simulink model "Model2_2023b"  (R2023b)
settings: Solver=ode4  StartTime=0.0  StopTime=100  FixedStep=0.01  RelTol=1e-3
values from neighbouring files (symbols this model uses):
  ARM_P_PID = [10 0 20]*0.1    [Single_ARM_Monte.m]    (also in main_starter.m)
  ARM_T_PID = [100 0 0]    [Single_ARM_Monte.m]    (also in main_starter.m)
  ARM_V_PID = [10 0 5]*0.1    [Single_ARM_Monte.m]    (also in main_starter.m)
  D_Joint0_angle0 = 45    [Single_ARM_Monte.m]    (also in main_starter.m)
  D_Joint0_angle1 = 0    [Single_ARM_Monte.m]    (also in main_starter.m)
  D_Joint0_angle2 = 0    [Single_ARM_Monte.m]    (also in main_starter.m)
  D_Joint0_rate0 = 0    [Single_ARM_Monte.m]    (also in main_starter.m)
  D_Joint0_rate1 = 0    [Single_ARM_Monte.m]    (also in main_starter.m)
  D_Joint0_rate2 = 0    [Single_ARM_Monte.m]    (also in main_starter.m)
  Joint_Motor_Mass = 23    [Single_ARM_Monte.m]    (also in main_starter.m)
  L_Joint0_angle0 = 45    [Single_ARM_Monte.m]    (also in main_starter.m)
  L_Joint0_angle1 = 0    [Single_ARM_Monte.m]    (also in main_starter.m)
  L_Joint0_angle2 = 0    [Single_ARM_Monte.m]    (also in main_starter.m)
  L_Joint0_rate0 = 0    [Single_ARM_Monte.m]    (also in main_starter.m)
  L_Joint0_rate1 = 0    [Single_ARM_Monte.m]    (also in main_starter.m)
  L_Joint0_rate2 = 0    [Single_ARM_Monte.m]    (also in main_starter.m)
  L_Joint_Offset = [ ... (first row only)    [Single_ARM_Monte.m]    (also in main_starter.m)
  Link1_Mass = 11    [Single_ARM_Monte.m]    (also in main_starter.m)
  Link2_Mass = 15.6    [Single_ARM_Monte.m]    (also in main_starter.m)
  Link3_Mass = 11    [Single_ARM_Monte.m]    (also in main_starter.m)
  Motor_transfer_Den = [1 100]    [Single_ARM_Monte.m]    (also in main_starter.m)
  Motor_transfer_Num = [100]    [Single_ARM_Monte.m]    (also in main_starter.m)
  PID_dt = 0.01    [Single_ARM_Monte.m]    (also in main_starter.m)
  R_Joint0_angle0 = 45    [Single_ARM_Monte.m]    (also in main_starter.m)
  R_Joint0_angle1 = 0    [Single_ARM_Monte.m]    (also in main_starter.m)
  R_Joint0_angle2 = 0    [Single_ARM_Monte.m]    (also in main_starter.m)
  R_Joint0_rate0 = 0    [Single_ARM_Monte.m]    (also in main_starter.m)
  R_Joint0_rate1 = 0    [Single_ARM_Monte.m]    (also in main_starter.m)
  R_Joint0_rate2 = 0    [Single_ARM_Monte.m]    (also in main_starter.m)
  RW_Att_D = 0.5    [Single_ARM_Monte.m]    (also in main_starter.m)
  RW_Att_I = 0.2    [Single_ARM_Monte.m]    (also in main_starter.m)
  RW_Att_P = 0.1    [Single_ARM_Monte.m]    (also in main_starter.m)
  RW_Mass = 100    [Single_ARM_Monte.m]    (also in main_starter.m)
  S_Body_Mass = 5    [Single_ARM_Monte.m]    (also in main_starter.m)
  S_init_pos = [0 0 0]'    [Single_ARM_Monte.m]    (also in main_starter.m)
  S_init_vel = [0 0 0]'    [Single_ARM_Monte.m]    (also in main_starter.m)
  T_Body_Mass = 4    [Single_ARM_Monte.m]    (also in main_starter.m)
  T_init_pos = [T_init_pos_list(i,1) T_init_pos_list(i,2) 0]'    [Single_ARM_Monte.m]    (also in main_starter.m = [1 0 0]')
  T_init_vel = [0 0 0]'    [Single_ARM_Monte.m]    (also in main_starter.m)
  Torq_mea_transfer_Den = [1 5]    [Single_ARM_Monte.m]    (also in main_starter.m)
  Torq_mea_transfer_Num = [5]    [Single_ARM_Monte.m]    (also in main_starter.m)
  U_Joint0_angle0 = 45    [Single_ARM_Monte.m]    (also in main_starter.m)
  U_Joint0_angle1 = 0    [Single_ARM_Monte.m]    (also in main_starter.m)
  U_Joint0_angle2 = 0    [Single_ARM_Monte.m]    (also in main_starter.m)
  U_Joint0_rate0 = 0    [Single_ARM_Monte.m]    (also in main_starter.m)
  U_Joint0_rate1 = 0    [Single_ARM_Monte.m]    (also in main_starter.m)
  U_Joint0_rate2 = 0    [Single_ARM_Monte.m]    (also in main_starter.m)
undefined symbols (not defined in the file or in its folder): X, Y, Z
libraries: nesl_utility x315, sm_lib x282, simulink_extras x46, sharedtransform x25, aerolibutil x4, simulink x2, matrix_library x2, dspmtrx3 x1
(part 2 of 12)

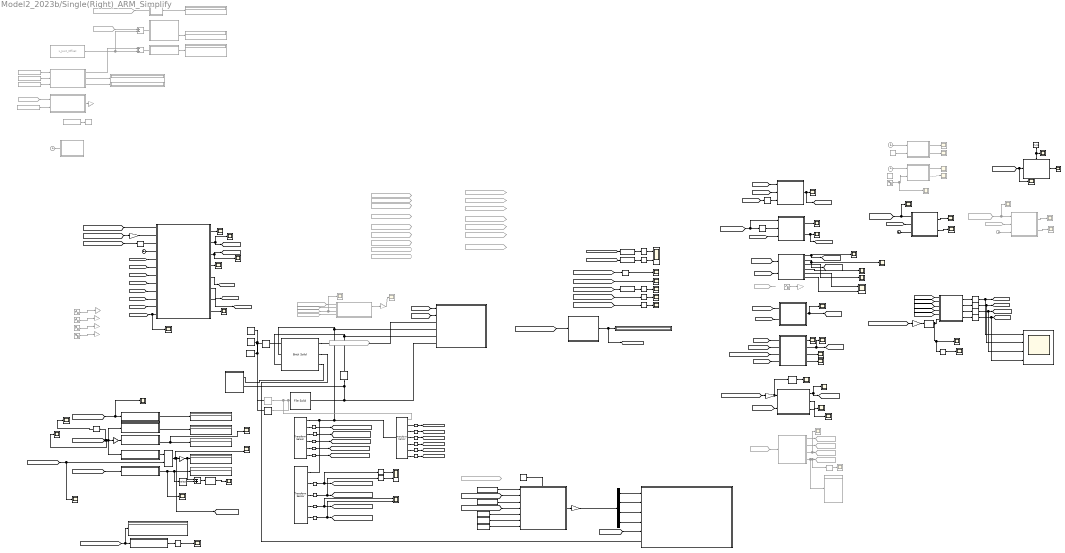
== system Model2_2023b/Single(Right)_ARM_Simplify ==
  note: 제어 명령을 맊으로 빼는 블럭
  note: Joint Translational Position, Velocity, Acceleration wrt Satellite Body
  note: Joint Translational Position, Velocity, Acceleration wrt Mount
  note: Each Link of Right ARM contact flag
  note: Right ARM Joint Angle, Rate, Accel
  note: Right ARM Joint Torque
  note: Relative Attitude with Target
  note: Angular Rate of Satellite wrt Body
  note: Angular Accel of Satellite wrt Body
  note: Relative Angular Rate with Target
  note: Attitude of Satellite Body wrt Iner
  6-DOF Joint1 : sm_lib/Joints/6-DOF Joint  Commented=on  JointMode=Normal  CompositeWrenchDir=FollowerOnBase  CompositeWrenchFrame=BaseFrame  SenseConstraintForce=off  SenseConstraintTorque=off  SenseTotalForce=off  SenseTotalTorque=off  PxPositionTargetSpecify=on  PxPositionTargetPriority=High  PxPositionTargetValue=0.3  PxPositionTargetValueUnits=m  PxVelocityTargetSpecify=on  PxVelocityTargetPriority=High  PxVelocityTargetValue=T_init_vel(1)  PxVelocityTargetValueUnits=m/s  PxEquilibriumPosition=0  PxEquilibriumPositionUnits=m  PxSpringStiffness=0  PxSpringStiffnessUnits=N/m  PxDampingCoefficient=0  PxDampingCoefficientUnits=N/(m/s)  PxLowerLimitSpecify=off  PxLowerLimitBound=-1  PxLowerLimitBoundUnits=m  PxLowerLimitStiffness=1e6  PxLowerLimitStiffnessUnits=N/m  PxLowerLimitDamping=1e3  PxLowerLimitDampingUnits=N/(m/s)  PxLowerLimitTransitionRegionWidth=1e-4  PxLowerLimitTransitionRegionWidthUnits=m  PxUpperLimitSpecify=off  PxUpperLimitBound=1  PxUpperLimitBoundUnits=m  PxUpperLimitStiffness=1e6  PxUpperLimitStiffnessUnits=N/m  PxUpperLimitDamping=1e3  PxUpperLimitDampingUnits=N/(m/s)  PxUpperLimitTransitionRegionWidth=1e-4  PxUpperLimitTransitionRegionWidthUnits=m  PxTorqueActuationMode=NoTorque  PxMotionActuationMode=ComputedMotion  PxSensePosition=off  PxSenseVelocity=off  PxSenseAcceleration=off  PxSenseTorqueForce=off  PxSenseLowerLimitTorqueForce=off  PxSenseUpperLimitTorqueForce=off  PyPositionTargetSpecify=on  PyPositionTargetPriority=High  PyPositionTargetValue=-0.01  PyPositionTargetValueUnits=m  PyVelocityTargetSpecify=on  PyVelocityTargetPriority=High  PyVelocityTargetValue=T_init_vel(2)  PyVelocityTargetValueUnits=m/s  PyEquilibriumPosition=0  PyEquilibriumPositionUnits=m  PySpringStiffness=0  PySpringStiffnessUnits=N/m  PyDampingCoefficient=0  PyDampingCoefficientUnits=N/(m/s)  PyLowerLimitSpecify=off  PyLowerLimitBound=-1  PyLowerLimitBoundUnits=m  PyLowerLimitStiffness=1e6  PyLowerLimitStiffnessUnits=N/m  PyLowerLimitDamping=1e3  PyLowerLimitDampingUnits=N/(m/s)  PyLowerLimitTransitionRegionWidth=1e-4  PyLowerLimitTransitionRegionWidthUnits=m  PyUpperLimitSpecify=off  PyUpperLimitBound=1  PyUpperLimitBoundUnits=m  PyUpperLimitStiffness=1e6  PyUpperLimitStiffnessUnits=N/m  PyUpperLimitDamping=1e3  PyUpperLimitDampingUnits=N/(m/s)  PyUpperLimitTransitionRegionWidth=1e-4  PyUpperLimitTransitionRegionWidthUnits=m  PyTorqueActuationMode=NoTorque  PyMotionActuationMode=ComputedMotion  PySensePosition=off  PySenseVelocity=off  PySenseAcceleration=off  PySenseTorqueForce=off  PySenseLowerLimitTorqueForce=off  PySenseUpperLimitTorqueForce=off  PzPositionTargetSpecify=on  PzPositionTargetPriority=High  PzPositionTargetValue=T_init_pos(3)  PzPositionTargetValueUnits=m  PzVelocityTargetSpecify=on  PzVelocityTargetPriority=High  PzVelocityTargetValue=T_init_vel(3)  PzVelocityTargetValueUnits=m/s  PzEquilibriumPosition=0  PzEquilibriumPositionUnits=m  PzSpringStiffness=0  PzSpringStiffnessUnits=N/m  PzDampingCoefficient=0  PzDampingCoefficientUnits=N/(m/s)  PzLowerLimitSpecify=off  PzLowerLimitBound=-1  PzLowerLimitBoundUnits=m  PzLowerLimitStiffness=1e6  PzLowerLimitStiffnessUnits=N/m  PzLowerLimitDamping=1e3  PzLowerLimitDampingUnits=N/(m/s)  PzLowerLimitTransitionRegionWidth=1e-4  PzLowerLimitTransitionRegionWidthUnits=m  PzUpperLimitSpecify=off  PzUpperLimitBound=1  PzUpperLimitBoundUnits=m  PzUpperLimitStiffness=1e6  PzUpperLimitStiffnessUnits=N/m  PzUpperLimitDamping=1e3  PzUpperLimitDampingUnits=N/(m/s)  PzUpperLimitTransitionRegionWidth=1e-4  PzUpperLimitTransitionRegionWidthUnits=m  PzTorqueActuationMode=NoTorque  PzMotionActuationMode=ComputedMotion  PzSensePosition=off  PzSenseVelocity=off  PzSenseAcceleration=off  PzSenseTorqueForce=off  PzSenseLowerLimitTorqueForce=off  PzSenseUpperLimitTorqueForce=off  SphPositionTargetSpecify=on  SphPositionTargetPriority=High  SphPositionTargetRotationMethod=RotationSequence  SphPositionTargetFollAlignAxisA=+X  SphPositionTargetBaseAlignAxisA=+Y  SphPositionTargetFollAlignAxisB=+Y  SphPositionTargetBaseAlignAxisB=+Z  SphPositionTargetRotationStandardAxis=+Z  SphPositionTargetRotationAngle=0.0  SphPositionTargetRotationAngleUnits=deg  SphPositionTargetRotationArbitraryAxis=[0 0 1]  SphPositionTargetRotationSequenceAxes=FollowerAxes  SphPositionTargetRotationSequence=ZYX  SphPositionTargetRotationSequenceAngles=T_init_att  SphPositionTargetRotationSequenceAnglesUnits=deg  SphPositionTargetRotationMatrix=[1 0 0; 0 1 0; 0 0 1]  SphPositionTargetQuaternion=[1 0 0 0]  SphVelocityTargetSpecify=on  SphVelocityTargetPriority=High  SphVelocityTargetValue=T_init_rate  SphVelocityTargetValueUnits=deg/s  SphVelocityTargetInFollowerFrame=on  SphEqPosRotationMethod=None  SphEqPosFollAlignAxisA=+X  SphEqPosBaseAlignAxisA=+Y  SphEqPosFollAlignAxisB=+Y  SphEqPosBaseAlignAxisB=+Z  SphEqPosRotationStandardAxis=+Z  SphEqPosRotationAngle=0.0  SphEqPosRotationAngleUnits=deg  SphEqPosRotationArbitraryAxis=[0 0 1]  SphEqPosRotationSequenceAxes=FollowerAxes  SphEqPosRotationSequence=XYX  SphEqPosRotationSequenceAngles=[0 0 0]  SphEqPosRotationSequenceAnglesUnits=deg  SphEqPosRotationMatrix=[1 0 0; 0 1 0; 0 0 1]  SphEqPosQuaternion=[1 0 0 0]  SphSpringStiffness=0  SphSpringStiffnessUnits=N*m/deg  SphDampingCoefficient=0  SphDampingCoefficientUnits=N*m/(deg/s)  SphLowerLimitSpecify=off  SphLowerLimitBound=15  SphLowerLimitBoundUnits=deg  SphLowerLimitStiffness=1e4  SphLowerLimitStiffnessUnits=N*m/deg  SphLowerLimitDamping=10  SphLowerLimitDampingUnits=N*m/(deg/s)  SphLowerLimitTransitionRegionWidth=0.1  SphLowerLimitTransitionRegionWidthUnits=deg  SphUpperLimitSpecify=off  SphUpperLimitBound=45  SphUpperLimitBoundUnits=deg  SphUpperLimitStiffness=1e4  SphUpperLimitStiffnessUnits=N*m/deg  SphUpperLimitDamping=10  SphUpperLimitDampingUnits=N*m/(deg/s)  SphUpperLimitTransitionRegionWidth=0.1  SphUpperLimitTransitionRegionWidthUnits=deg  SphTorqueActuationMode=NoTorque  SphActuateTorqueX=off  SphActuateTorqueY=off  SphActuateTorqueZ=off  SphActuateTorque=off  SphActuationFrame=BaseFrame  SphSensePosition=off  SphSenseVelocityX=off  SphSenseVelocityY=off  SphSenseVelocityZ=off  SphSenseVelocity=off  SphSenseAccelerationX=off  SphSenseAccelerationY=off  SphSenseAccelerationZ=off  SphSenseAcceleration=off  SphSenseLowerLimitTorqueMag=off  SphSenseUpperLimitTorqueMag=off  SphSensingFrame=BaseFrame
  6-DOF Joint2 : sm_lib/Joints/6-DOF Joint  JointMode=Normal  CompositeWrenchDir=FollowerOnBase  CompositeWrenchFrame=BaseFrame  SenseConstraintForce=off  SenseConstraintTorque=off  SenseTotalForce=off  SenseTotalTorque=off  PxPositionTargetSpecify=on  PxPositionTargetPriority=High  PxPositionTargetValue=S_init_pos(1)  PxPositionTargetValueUnits=m  PxVelocityTargetSpecify=on  PxVelocityTargetPriority=High  PxVelocityTargetValue=S_init_vel(1)  PxVelocityTargetValueUnits=m/s  PxEquilibriumPosition=0  PxEquilibriumPositionUnits=m  PxSpringStiffness=0  PxSpringStiffnessUnits=N/m  PxDampingCoefficient=0  PxDampingCoefficientUnits=N/(m/s)  PxLowerLimitSpecify=off  PxLowerLimitBound=-1  PxLowerLimitBoundUnits=m  PxLowerLimitStiffness=1e6  PxLowerLimitStiffnessUnits=N/m  PxLowerLimitDamping=1e3  PxLowerLimitDampingUnits=N/(m/s)  PxLowerLimitTransitionRegionWidth=1e-4  PxLowerLimitTransitionRegionWidthUnits=m  PxUpperLimitSpecify=off  PxUpperLimitBound=1  PxUpperLimitBoundUnits=m  PxUpperLimitStiffness=1e6  PxUpperLimitStiffnessUnits=N/m  PxUpperLimitDamping=1e3  PxUpperLimitDampingUnits=N/(m/s)  PxUpperLimitTransitionRegionWidth=1e-4  PxUpperLimitTransitionRegionWidthUnits=m  PxTorqueActuationMode=NoTorque  PxMotionActuationMode=ComputedMotion  PxSensePosition=off  PxSenseVelocity=off  PxSenseAcceleration=off  PxSenseTorqueForce=off  PxSenseLowerLimitTorqueForce=off  PxSenseUpperLimitTorqueForce=off  PyPositionTargetSpecify=on  PyPositionTargetPriority=High  PyPositionTargetValue=S_init_pos(2)  PyPositionTargetValueUnits=m  PyVelocityTargetSpecify=on  PyVelocityTargetPriority=High  PyVelocityTargetValue=S_init_vel(2)  PyVelocityTargetValueUnits=m/s  PyEquilibriumPosition=0  PyEquilibriumPositionUnits=m  PySpringStiffness=0  PySpringStiffnessUnits=N/m  PyDampingCoefficient=0  PyDampingCoefficientUnits=N/(m/s)  PyLowerLimitSpecify=off  PyLowerLimitBound=-1  PyLowerLimitBoundUnits=m  PyLowerLimitStiffness=1e6  PyLowerLimitStiffnessUnits=N/m  PyLowerLimitDamping=1e3  PyLowerLimitDampingUnits=N/(m/s)  PyLowerLimitTransitionRegionWidth=1e-4  PyLowerLimitTransitionRegionWidthUnits=m  PyUpperLimitSpecify=off  PyUpperLimitBound=1  PyUpperLimitBoundUnits=m  PyUpperLimitStiffness=1e6  PyUpperLimitStiffnessUnits=N/m  PyUpperLimitDamping=1e3  PyUpperLimitDampingUnits=N/(m/s)  PyUpperLimitTransitionRegionWidth=1e-4  PyUpperLimitTransitionRegionWidthUnits=m  PyTorqueActuationMode=NoTorque  PyMotionActuationMode=ComputedMotion  PySensePosition=off  PySenseVelocity=off  PySenseAcceleration=off  PySenseTorqueForce=off  PySenseLowerLimitTorqueForce=off  PySenseUpperLimitTorqueForce=off  PzPositionTargetSpecify=on  PzPositionTargetPriority=High  PzPositionTargetValue=S_init_pos(3)  PzPositionTargetValueUnits=m  PzVelocityTargetSpecify=on  PzVelocityTargetPriority=High  PzVelocityTargetValue=S_init_vel(3)  PzVelocityTargetValueUnits=m/s  PzEquilibriumPosition=0  PzEquilibriumPositionUnits=m  PzSpringStiffness=0  PzSpringStiffnessUnits=N/m  PzDampingCoefficient=0  PzDampingCoefficientUnits=N/(m/s)  PzLowerLimitSpecify=off  PzLowerLimitBound=-1  PzLowerLimitBoundUnits=m  PzLowerLimitStiffness=1e6  PzLowerLimitStiffnessUnits=N/m  PzLowerLimitDamping=1e3  PzLowerLimitDampingUnits=N/(m/s)  PzLowerLimitTransitionRegionWidth=1e-4  PzLowerLimitTransitionRegionWidthUnits=m  PzUpperLimitSpecify=off  PzUpperLimitBound=1  PzUpperLimitBoundUnits=m  PzUpperLimitStiffness=1e6  PzUpperLimitStiffnessUnits=N/m  PzUpperLimitDamping=1e3  PzUpperLimitDampingUnits=N/(m/s)  PzUpperLimitTransitionRegionWidth=1e-4  PzUpperLimitTransitionRegionWidthUnits=m  PzTorqueActuationMode=NoTorque  PzMotionActuationMode=ComputedMotion  PzSensePosition=off  PzSenseVelocity=off  PzSenseAcceleration=off  PzSenseTorqueForce=off  PzSenseLowerLimitTorqueForce=off  PzSenseUpperLimitTorqueForce=off  SphPositionTargetSpecify=on  SphPositionTargetPriority=High  SphPositionTargetRotationMethod=RotationSequence  SphPositionTargetFollAlignAxisA=+X  SphPositionTargetBaseAlignAxisA=+Y  SphPositionTargetFollAlignAxisB=+Y  SphPositionTargetBaseAlignAxisB=+Z  SphPositionTargetRotationStandardAxis=+Z  SphPositionTargetRotationAngle=0.0  SphPositionTargetRotationAngleUnits=deg  SphPositionTargetRotationArbitraryAxis=[0 0 1]  SphPositionTargetRotationSequenceAxes=FollowerAxes  SphPositionTargetRotationSequence=ZYX  SphPositionTargetRotationSequenceAngles=S_init_att  SphPositionTargetRotationSequenceAnglesUnits=deg  SphPositionTargetRotationMatrix=[1 0 0; 0 1 0; 0 0 1]  SphPositionTargetQuaternion=[1 0 0 0]  SphVelocityTargetSpecify=on  SphVelocityTargetPriority=High  SphVelocityTargetValue=S_init_rate  SphVelocityTargetValueUnits=deg/s  SphVelocityTargetInFollowerFrame=on  SphEqPosRotationMethod=None  SphEqPosFollAlignAxisA=+X  SphEqPosBaseAlignAxisA=+Y  SphEqPosFollAlignAxisB=+Y  SphEqPosBaseAlignAxisB=+Z  SphEqPosRotationStandardAxis=+Z  SphEqPosRotationAngle=0.0  SphEqPosRotationAngleUnits=deg  SphEqPosRotationArbitraryAxis=[0 0 1]  SphEqPosRotationSequenceAxes=FollowerAxes  SphEqPosRotationSequence=XYX  SphEqPosRotationSequenceAngles=[0 0 0]  SphEqPosRotationSequenceAnglesUnits=deg  SphEqPosRotationMatrix=[1 0 0; 0 1 0; 0 0 1]  SphEqPosQuaternion=[1 0 0 0]  SphSpringStiffness=0  SphSpringStiffnessUnits=N*m/deg  SphDampingCoefficient=0  SphDampingCoefficientUnits=N*m/(deg/s)  SphLowerLimitSpecify=off  SphLowerLimitBound=15  SphLowerLimitBoundUnits=deg  SphLowerLimitStiffness=1e4  SphLowerLimitStiffnessUnits=N*m/deg  SphLowerLimitDamping=10  SphLowerLimitDampingUnits=N*m/(deg/s)  SphLowerLimitTransitionRegionWidth=0.1  SphLowerLimitTransitionRegionWidthUnits=deg  SphUpperLimitSpecify=off  SphUpperLimitBound=45  SphUpperLimitBoundUnits=deg  SphUpperLimitStiffness=1e4  SphUpperLimitStiffnessUnits=N*m/deg  SphUpperLimitDamping=10  SphUpperLimitDampingUnits=N*m/(deg/s)  SphUpperLimitTransitionRegionWidth=0.1  SphUpperLimitTransitionRegionWidthUnits=deg  SphTorqueActuationMode=NoTorque  SphActuateTorqueX=off  SphActuateTorqueY=off  SphActuateTorqueZ=off  SphActuateTorque=off  SphActuationFrame=BaseFrame  SphSensePosition=off  SphSenseVelocityX=off  SphSenseVelocityY=off  SphSenseVelocityZ=off  SphSenseVelocity=off  SphSenseAccelerationX=off  SphSenseAccelerationY=off  SphSenseAccelerationZ=off  SphSenseAcceleration=off  SphSenseLowerLimitTorqueMag=off  SphSenseUpperLimitTorqueMag=off  SphSensingFrame=BaseFrame
  6-DOF Joint3 : sm_lib/Joints/6-DOF Joint  JointMode=Normal  CompositeWrenchDir=FollowerOnBase  CompositeWrenchFrame=BaseFrame  SenseConstraintForce=off  SenseConstraintTorque=off  SenseTotalForce=off  SenseTotalTorque=off  PxPositionTargetSpecify=on  PxPositionTargetPriority=High  PxPositionTargetValue=0.35  PxPositionTargetValueUnits=m  PxVelocityTargetSpecify=on  PxVelocityTargetPriority=High  PxVelocityTargetValue=T_init_vel(1)  PxVelocityTargetValueUnits=m/s  PxEquilibriumPosition=0  PxEquilibriumPositionUnits=m  PxSpringStiffness=0  PxSpringStiffnessUnits=N/m  PxDampingCoefficient=0  PxDampingCoefficientUnits=N/(m/s)  PxLowerLimitSpecify=off  PxLowerLimitBound=-1  PxLowerLimitBoundUnits=m  PxLowerLimitStiffness=1e6  PxLowerLimitStiffnessUnits=N/m  PxLowerLimitDamping=1e3  PxLowerLimitDampingUnits=N/(m/s)  PxLowerLimitTransitionRegionWidth=1e-4  PxLowerLimitTransitionRegionWidthUnits=m  PxUpperLimitSpecify=off  PxUpperLimitBound=1  PxUpperLimitBoundUnits=m  PxUpperLimitStiffness=1e6  PxUpperLimitStiffnessUnits=N/m  PxUpperLimitDamping=1e3  PxUpperLimitDampingUnits=N/(m/s)  PxUpperLimitTransitionRegionWidth=1e-4  PxUpperLimitTransitionRegionWidthUnits=m  PxTorqueActuationMode=NoTorque  PxMotionActuationMode=ComputedMotion  PxSensePosition=off  PxSenseVelocity=off  PxSenseAcceleration=off  PxSenseTorqueForce=off  PxSenseLowerLimitTorqueForce=off  PxSenseUpperLimitTorqueForce=off  PyPositionTargetSpecify=on  PyPositionTargetPriority=High  PyPositionTargetValue=0.09  PyPositionTargetValueUnits=m  PyVelocityTargetSpecify=on  PyVelocityTargetPriority=High  PyVelocityTargetValue=T_init_vel(2)  PyVelocityTargetValueUnits=m/s  PyEquilibriumPosition=0  PyEquilibriumPositionUnits=m  PySpringStiffness=0  PySpringStiffnessUnits=N/m  PyDampingCoefficient=0  PyDampingCoefficientUnits=N/(m/s)  PyLowerLimitSpecify=off  PyLowerLimitBound=-1  PyLowerLimitBoundUnits=m  PyLowerLimitStiffness=1e6  PyLowerLimitStiffnessUnits=N/m  PyLowerLimitDamping=1e3  PyLowerLimitDampingUnits=N/(m/s)  PyLowerLimitTransitionRegionWidth=1e-4  PyLowerLimitTransitionRegionWidthUnits=m  PyUpperLimitSpecify=off  PyUpperLimitBound=1  PyUpperLimitBoundUnits=m  PyUpperLimitStiffness=1e6  PyUpperLimitStiffnessUnits=N/m  PyUpperLimitDamping=1e3  PyUpperLimitDampingUnits=N/(m/s)  PyUpperLimitTransitionRegionWidth=1e-4  PyUpperLimitTransitionRegionWidthUnits=m  PyTorqueActuationMode=NoTorque  PyMotionActuationMode=ComputedMotion  PySensePosition=off  PySenseVelocity=off  PySenseAcceleration=off  PySenseTorqueForce=off  PySenseLowerLimitTorqueForce=off  PySenseUpperLimitTorqueForce=off  PzPositionTargetSpecify=on  PzPositionTargetPriority=High  PzPositionTargetValue=T_init_pos(3)  PzPositionTargetValueUnits=m  PzVelocityTargetSpecify=on  PzVelocityTargetPriority=High  PzVelocityTargetValue=T_init_vel(3)  PzVelocityTargetValueUnits=m/s  PzEquilibriumPosition=0  PzEquilibriumPositionUnits=m  PzSpringStiffness=0  PzSpringStiffnessUnits=N/m  PzDampingCoefficient=0  PzDampingCoefficientUnits=N/(m/s)  PzLowerLimitSpecify=off  PzLowerLimitBound=-1  PzLowerLimitBoundUnits=m  PzLowerLimitStiffness=1e6  PzLowerLimitStiffnessUnits=N/m  PzLowerLimitDamping=1e3  PzLowerLimitDampingUnits=N/(m/s)  PzLowerLimitTransitionRegionWidth=1e-4  PzLowerLimitTransitionRegionWidthUnits=m  PzUpperLimitSpecify=off  PzUpperLimitBound=1  PzUpperLimitBoundUnits=m  PzUpperLimitStiffness=1e6  PzUpperLimitStiffnessUnits=N/m  PzUpperLimitDamping=1e3  PzUpperLimitDampingUnits=N/(m/s)  PzUpperLimitTransitionRegionWidth=1e-4  PzUpperLimitTransitionRegionWidthUnits=m  PzTorqueActuationMode=NoTorque  PzMotionActuationMode=ComputedMotion  PzSensePosition=off  PzSenseVelocity=off  PzSenseAcceleration=off  PzSenseTorqueForce=off  PzSenseLowerLimitTorqueForce=off  PzSenseUpperLimitTorqueForce=off  SphPositionTargetSpecify=on  SphPositionTargetPriority=High  SphPositionTargetRotationMethod=RotationSequence  SphPositionTargetFollAlignAxisA=+X  SphPositionTargetBaseAlignAxisA=+Y  SphPositionTargetFollAlignAxisB=+Y  SphPositionTargetBaseAlignAxisB=+Z  SphPositionTargetRotationStandardAxis=+Z  SphPositionTargetRotationAngle=0.0  SphPositionTargetRotationAngleUnits=deg  SphPositionTargetRotationArbitraryAxis=[0 0 1]  SphPositionTargetRotationSequenceAxes=FollowerAxes  SphPositionTargetRotationSequence=ZYX  SphPositionTargetRotationSequenceAngles=T_init_att  SphPositionTargetRotationSequenceAnglesUnits=deg  SphPositionTargetRotationMatrix=[1 0 0; 0 1 0; 0 0 1]  SphPositionTargetQuaternion=[1 0 0 0]  SphVelocityTargetSpecify=on  SphVelocityTargetPriority=High  SphVelocityTargetValue=[0 0 0]  SphVelocityTargetValueUnits=deg/s  SphVelocityTargetInFollowerFrame=on  SphEqPosRotationMethod=None  SphEqPosFollAlignAxisA=+X  SphEqPosBaseAlignAxisA=+Y  SphEqPosFollAlignAxisB=+Y  SphEqPosBaseAlignAxisB=+Z  SphEqPosRotationStandardAxis=+Z  SphEqPosRotationAngle=0.0  SphEqPosRotationAngleUnits=deg  SphEqPosRotationArbitraryAxis=[0 0 1]  SphEqPosRotationSequenceAxes=FollowerAxes  SphEqPosRotationSequence=XYX  SphEqPosRotationSequenceAngles=[0 0 0]  SphEqPosRotationSequenceAnglesUnits=deg  SphEqPosRotationMatrix=[1 0 0; 0 1 0; 0 0 1]  SphEqPosQuaternion=[1 0 0 0]  SphSpringStiffness=0  SphSpringStiffnessUnits=N*m/deg  SphDampingCoefficient=0  SphDampingCoefficientUnits=N*m/(deg/s)  SphLowerLimitSpecify=off  SphLowerLimitBound=15  SphLowerLimitBoundUnits=deg  SphLowerLimitStiffness=1e4  SphLowerLimitStiffnessUnits=N*m/deg  SphLowerLimitDamping=10  SphLowerLimitDampingUnits=N*m/(deg/s)  SphLowerLimitTransitionRegionWidth=0.1  SphLowerLimitTransitionRegionWidthUnits=deg  SphUpperLimitSpecify=off  SphUpperLimitBound=45  SphUpperLimitBoundUnits=deg  SphUpperLimitStiffness=1e4  SphUpperLimitStiffnessUnits=N*m/deg  SphUpperLimitDamping=10  SphUpperLimitDampingUnits=N*m/(deg/s)  SphUpperLimitTransitionRegionWidth=0.1  SphUpperLimitTransitionRegionWidthUnits=deg  SphTorqueActuationMode=NoTorque  SphActuateTorqueX=off  SphActuateTorqueY=off  SphActuateTorqueZ=off  SphActuateTorque=off  SphActuationFrame=BaseFrame  SphSensePosition=off  SphSenseVelocityX=off  SphSenseVelocityY=off  SphSenseVelocityZ=off  SphSenseVelocity=off  SphSenseAccelerationX=off  SphSenseAccelerationY=off  SphSenseAccelerationZ=off  SphSenseAcceleration=off  SphSenseLowerLimitTorqueMag=off  SphSenseUpperLimitTorqueMag=off  SphSensingFrame=BaseFrame
  Add : Sum  Inputs=-+
  Add3 : Sum  Commented=on
  Add5 : Sum  Commented=on  Inputs=+-
  Attitude:Rel,Iner : Scope  NumInputPorts=2
  Attitude_iner[deg] : Scope
  Brick Solid : sm_lib/Body Elements/Brick Solid  BrickDimensions=[30 30 40]  BrickDimensionsUnits=cm  ExportEntireGeometry=on  InertiaType=CalculateFromGeometry  BasedOnType=Mass  Density=1000  DensityUnits=kg/m^3  Mass=S_Body_Mass  MassUnits=kg  CenterOfMass=[0 0 0]  CenterOfMassUnits=m  MomentsOfInertia=[1 1 1]  MomentsOfInertiaUnits=kg*m^2  ProductsOfInertia=[0 0 0]  ProductsOfInertiaUnits=kg*m^2  GraphicType=FromGeometry  MarkerShape=Sphere  MarkerSize=10  GraphicVisPropType=SimpleVisualProperties  GraphicDiffuseColor=[0.4 0.4 0.4]  GraphicOpacity=0.2  GraphicSpecularColor=[0.5 0.5 0.5 1.0]  GraphicAmbientColor=[0.15 0.15 0.15 1.0]  GraphicEmissiveColor=[0.0 0.0 0.0 1.0]  GraphicShininess=75  DoExposeReferenceFrame=on  SerializedFrames=<Frames><Frame><Id>Frame2</Id><Value><Name>Right_ARM_F</Name><Origin><Source>ReferenceFrame</Source><FeatureName></FeatureName></Origin><PrimaryAxis><DefinedDirection>+Z</DefinedDirection><Source>ReferenceFrame</Source><SourceDirection>+Z</SourceDirection><FeatureName></FeatureName></PrimaryAxis><SecondaryAxis><DefinedDirection>+X</DefinedDirection><Source>ReferenceFrame</Source><SourceDirection>+X</SourceDirection><FeatureName></FeatureName></SecondaryAxis></Value></Frame><Frame><Id>Frame3</Id><Value><Name>RW_F</Name><Origin><Source>CenterOfMassFrame</Source><FeatureName></FeatureName></Origin><PrimaryAxis><DefinedDirection>+Z</DefinedDirection><Source>ReferenceFrame</Source><SourceDirection>+Z</SourceDirection><FeatureName></FeatureName></PrimaryAxis><SecondaryAxis><DefinedDirection>+X</DefinedDirection><Source>ReferenceFrame</Source><SourceDirection>+X</SourceDirection><FeatureName></FeatureName></SecondaryAxis></Value></Frame><Frame><Id>Frame4</Id><Value><Name>CoM_F</Name><Origin><Source>ReferenceFrame</Source><FeatureName></FeatureName></Origin><PrimaryAxis><DefinedDirection>+Z</DefinedDirection><Source>ReferenceFrame</Source><SourceDirection>+Z</SourceDirection><FeatureName></FeatureName></PrimaryAxis><SecondaryAxis><DefinedDirection>+X</DefinedDirection><Source>ReferenceFrame</Source><SourceDirection>+X</SourceDirection><FeatureName></FeatureName></SecondaryAxis></Value></Frame><Frame><Id>Frame5</Id><Value><Name>Body_Contact_Sensor_F</Name><Origin><Source>GeometricFeature</Source><FeatureName>+x surface</FeatureName></Origin><PrimaryAxis><DefinedDirection>+Z</DefinedDirection><Source>ReferenceFrame</Source><SourceDirection>+Z</SourceDirection><FeatureName></FeatureName></PrimaryAxis><SecondaryAxis><DefinedDirection>+X</DefinedDirection><Source>ReferenceFrame</Source><SourceDirection>+X</SourceDirection><FeatureName></FeatureName></SecondaryAxis></Value></Frame></Frames>
  Clock : Clock
  Clock{1..2,4..5} (4 alike) : Clock  Commented=on
  Clock3 : Clock
  Constant : Constant  Commented=on  Value=L_Joint_Offset
  Constant1 : Constant  Value=[0 0 0]'
  Constant10 : Constant  Value=RW_Att_D
  Constant2 : Constant  Commented=on  Value=[0.3 0.3]'
  Constant3 : Constant  Commented=on  Value=[0.3 0.3]'
  Constant4 : Constant  Commented=on  Value=0.001
  Constant5 : Constant  Commented=on  Value=100
  Constant6 : Constant  Commented=on  Value=[45 -90 -180]'
  Constant7 : Constant  Value=[0 0 0]'
  Constant8 : Constant  Value=RW_Att_P
  Constant9 : Constant  Value=RW_Att_I
  Degrees to Radians : simulink_extras/Transformations/Degrees to Radians  Commented=on
  Delay : Delay  DelayLength=300
  Delay{1..5} (5 alike) : Delay  DelayLength=1
  Demux1 : Demux
  Derivative : Derivative
  Derivative1 : Derivative  Commented=on
  Derivative3 : Derivative
  Derivative4 : Derivative
  Display{,1..2,4,6..7} (6 alike) : Display  Commented=on
  Display{3,8,13..14,16..18} (7 alike) : Display
  EE_R : MATLAB Function  Commented=on  TreatAsAtomicUnit=on
  Empty : MATLAB Function  TreatAsAtomicUnit=on
  End_Position_Flg : MATLAB Function  TreatAsAtomicUnit=on
  Fabrik_based_EE_Control(Angle) : MATLAB Function  Commented=on  TreatAsAtomicUnit=on
  From102 : From  Commented=on  GotoTag=R_J
  From12 : From  Commented=on  GotoTag=Right_ARM_J  TagVisibility=global
  From13 : From  Commented=on  GotoTag=Right_ARM_J_Pos_Mount  TagVisibility=global
  From14 : From  Commented=on  GotoTag=Right_ARM_Jt  TagVisibility=global
  From16 : From  Commented=on  GotoTag=Relative_quat
  From19 : From  Commented=on  GotoTag=S_Rate_wrt_Body  TagVisibility=global
  From2 : From  Commented=on  GotoTag=ARM_J  TagVisibility=global
  From20 : From  Commented=on  GotoTag=B_f_contact  TagVisibility=global
  From22 : From  Commented=on  GotoTag=S_Rated_wrt_Body  TagVisibility=global
  From23 : From  Commented=on  GotoTag=Relative_quat
  From24 : From  Commented=on  GotoTag=Right_ARM_Jd  TagVisibility=global
  From25 : From  Commented=on  GotoTag=Right_ARM_Jdd  TagVisibility=global
  From26 : From  Commented=on  GotoTag=Right_ARM_J_Pos_SB  TagVisibility=global
  From27 : From  Commented=on  GotoTag=Right_ARM_J_Vel_SB  TagVisibility=global
  From3 : From  Commented=on  GotoTag=LEFT_ARM_J_Pos_Mount
  From31 : From  Commented=on  GotoTag=Right_ARM_J_Acc_SB  TagVisibility=global
  From32 : From  Commented=on  GotoTag=Pos_END_FLAG
  From33 : From  Commented=on  GotoTag=Right_ARM_J_Pos_Mount  TagVisibility=global
  From34 : From  Commented=on  GotoTag=Right_ARM_J_Vel_Mount  TagVisibility=global
  From35 : From  Commented=on  GotoTag=Right_ARM_J_Acc_Mount  TagVisibility=global
  From36 : From  Commented=on  GotoTag=Right_ARM_Link_Contact_flg  TagVisibility=global
  From37 : From  Commented=on  GotoTag=Relative_w
  From38 : From  Commented=on  GotoTag=Right_ARM_J_Pos_Mount  TagVisibility=global
  From4 : From  Commented=on  GotoTag=LEFT_ARM_J
  From41 : From  Commented=on  GotoTag=slip_start
  From7 : From  Commented=on  GotoTag=S_Attitude_quat_Inertial  TagVisibility=global
  From78 : From  Commented=on  GotoTag=EE_Jaco_start
  From79 : From  Commented=on  GotoTag=EE_vel_J
  From9 : From  Commented=on  GotoTag=Right_ARM_J  TagVisibility=global
  Gain : Gain  Commented=on
  Gain1 : Gain  Gain=100
  Gain2 : Gain
  Gain3 : Gain  Gain=100
  Gain4 : Gain  Gain=100
  Gain7 : Gain
  Gain8 : Gain
  Gain9 : Gain  Commented=on
  Goto49 : Goto  Commented=on  GotoTag=RPos_0
  Goto50 : Goto  Commented=on  GotoTag=RPos_1
  Goto51 : Goto  Commented=on  GotoTag=RPos_2
  Goto52 : Goto  Commented=on  GotoTag=RPos_3
  Jacobian_based_EE_Control(Rate) : MATLAB Function  Commented=on  TreatAsAtomicUnit=on
  MATLAB Function : MATLAB Function  Commented=on  TreatAsAtomicUnit=on
  MATLAB Function1 : MATLAB Function  TreatAsAtomicUnit=on
  MATLAB Function11 : MATLAB Function  TreatAsAtomicUnit=on
  MATLAB Function16 : MATLAB Function  TreatAsAtomicUnit=on
  MATLAB Function2 : MATLAB Function  Commented=on  TreatAsAtomicUnit=on
  MATLAB Function3 : MATLAB Function  TreatAsAtomicUnit=on
  MATLAB Function4 : MATLAB Function  TreatAsAtomicUnit=on
  MATLAB Function5 : MATLAB Function  Commented=on  TreatAsAtomicUnit=on
  MATLAB Function6 : MATLAB Function  Commented=on  TreatAsAtomicUnit=on
  MATLAB Function7 : MATLAB Function  Commented=on  TreatAsAtomicUnit=on
  Matrix 1-Norm : dspmtrx3/Matrix  1-Norm  roundingMode=Floor  overflowMode=off  outputDataTypeStr=Inherit: Same as accumulator  outputMin=[]  outputMax=[]  outputLastDataTypeStr=Inherit: Same as accumulator
  Matrix Multiply1 : Product  Multiplication=Matrix(*)
  Mechanism Configuration : sm_lib/Utilities/Mechanism Configuration  UniformGravity=None  GravityVector=[0 0 -9.80665]  GravityVectorUnits=m/s^2  LinearizationDelta=0.001  JointModeTransitionNonlinearIterations=2
  Multiply{,1..4} (5 alike) : Gain  Commented=on  Gain=0
  Openning_Motion_Sequence1 : MATLAB Function  Commented=on  TreatAsAtomicUnit=on
  Openning_Motion_Sequence4 : MATLAB Function  Commented=on  TreatAsAtomicUnit=on
  Overload : MATLAB Function  TreatAsAtomicUnit=on
  PS-Simulink Converter{1..7,13..15,23,26..28,38} (15 alike) : nesl_utility/PS-Simulink Converter  PhysicalDomain=network_engine_domain  SubClassName=ps_output  LeftPortType=input  RightPortType=output  PseudoPeriodic=off  Frequencies=[]  VectorFormat=inherit  Unit=inherit  AffineConversion=off
  Pulse Generator : DiscretePulseGenerator  PulseType=Time based  Period=0.2  PulseWidth=50
  Pulse Generator1 : DiscretePulseGenerator  PulseType=Time based  Period=0.5  PulseWidth=50
  Quaternions to Rotation Angles : sharedtransform/Quaternions to Rotation Angles  rotationOrder=ZYX  aMode=aMode
  Quaternions to Rotation Angles1 : sharedtransform/Quaternions to Rotation Angles  rotationOrder=ZYX  aMode=aMode
  Quaternions to Rotation Angles2 : sharedtransform/Quaternions to Rotation Angles  rotationOrder=ZYX  aMode=aMode
  Radians to Degrees{,1..8} (9 alike) : simulink_extras/Transformations/Radians to Degrees
  Ramp : simulink/Sources/Ramp  Commented=on  slope=1.4  start=0  InitialOutput=0
  Ramp2 : simulink/Sources/Ramp  Commented=on  slope=1  start=0  InitialOutput=0
  Right_ARM : Subsystem
  Right_ARM_Jacobian : MATLAB Function  TreatAsAtomicUnit=on
  Right_ARM_Real_FK : MATLAB Function  TreatAsAtomicUnit=on
  Right_ARM_Real_Simple_FK : MATLAB Function  TreatAsAtomicUnit=on
  Right_Joint_Angle[deg] : Scope
  Right_Joint_Torque[Nm] : Scope
  Scope{,1..4,6,9,11..13,15,17,19..28,30..33,35..36,38..42,45,52..54} (37 alike) : Scope
  Scope{8,10,16,18,43..44,46..51} (12 alike) : Scope  Commented=on
  Scope{5,7,14,29,34} (5 alike) : Scope  NumInputPorts=2
  Scope37 : Scope  NumInputPorts=4
  Selector : Selector  InputPortWidth=3  IndexOptions=Index vector (dialog)  Indices=[1 2]  OutputSizes=1
  Sine Wave{,1..5} (6 alike) : Sin  Commented=on  SampleTime=0
  Slip_current : MATLAB Function  TreatAsAtomicUnit=on
  Solver Configuration : nesl_utility/Solver Configuration  PhysicalDomain=network_engine_domain  SubClassName=solver  LeftPortType=input  RightPortType=generic  Tones=[]  Harmonics=[]  SimulateNoise=off  Profile=off  UseLocalSampling=off  EnableSwitchedLinearOptims=on  FrequencyDomain=off  UseCCode=off  RelTol=0.001  AbsTol=0.001  MinStep=1e-09  ToWorkspace=off  RevertToSquareIcSolve=off  NumHomotopyIterations=100  PhasorMode=off  PhasorModeNumHarmonics=1  ConsistencySolver=NEWTON_XTOL_AFTER_FTOL  IndexReductionMethod=DerivativeReplacement  DoDC=off  ResidualTolerance=1e-09  ConsistencyTolSource=GLOBAL  ConsistencyAbsTol=0.001  ConsistencyRelTol=0.001  ConsistencyTolFactor=0.001  UseLocalSolver=off  LocalSolverChoice=NE_BACKWARD_EULER_ADVANCER  ResolveIndetEquations=on  FunctionEvalNumThread=1  LocalSolverSampleTime=0.001  DoFixedCost=off  MaxNonlinIter=3  MaxModeIter=2  ComputeImpulses=off  ImpulseIterations=2  LinearAlgebra=auto  LinearAlgebraNumThread=0  EquationFormulation=NE_TIME_EF  DelaysMemoryBudget=1024  AutomaticFiltering=on  FilteringTimeConstant=0.001  PartitionStorageMethod=AS_NEEDED  PartitionMemoryBudget=1024  PartitionMethod=ROBUST  MultibodyUseLocalSolver=off  MultibodyLocalSolverChoice=ODE1  MultibodyLocalSolverSampleTime=0.001
  Spatial Contact Force6 : sm_lib/Forces and Torques/Spatial Contact Force  NormalForceType=SmoothSpringDamper  NormalStiffness=B2T_Siffness  NormalStiffnessUnits=N/m  NormalDamping=B2T_Damping  NormalDampingUnits=N/(m/s)  NormalTransitionRegionWidth=B2T_TRW  NormalTransitionRegionWidthUnits=m  FrictionType=SmoothStickSlip  CoefficientOfStaticFriction=0.8  CoefficientOfDynamicFriction=0.6  FrictionalCriticalVelocity=1e-3  FrictionalCriticalVelocityUnits=m/s  SenseContactSignal=off  SensePenetrationDepth=off  SenseSeparationDistance=off  SenseNormalForceMagnitude=off  SenseFrictionalForceMagnitude=off  SenseNormalVelocity=off  SenseTangentialVelocity=off  SenseContactBaseRotation=off  SenseContactBaseTranslation=off  SenseContactFollowerRotation=off  SenseContactFollowerTranslation=off  ZeroCrossDetectContactStartAndEnd=off
  Submatrix : matrix_library/Submatrix  RowSpan=All rows  RowStartMode=First  RowStartIndex=1  RowEndMode=Last  RowEndIndex=1  ColSpan=Range of columns  ColStartMode=Offset from last  ColStartIndex=0  ColEndMode=Last  ColEndIndex=1
  Submatrix1 : matrix_library/Submatrix  RowSpan=All rows  RowStartMode=First  RowStartIndex=1  RowEndMode=Last  RowEndIndex=1  ColSpan=Range of columns  ColStartMode=Offset from last  ColStartIndex=0  ColEndMode=Last  ColEndIndex=1
  Subsystem : Subsystem
  Subsystem1 : Subsystem
  Subsystem2 : Subsystem
  Subsystem5 : Subsystem
  Target : sm_lib/Body Elements/File Solid  ExtGeomFileName=../\target_model\cubesat_12_0U.stl  UnitType=Custom  ExtGeomFileUnits=mm  StepReaderType=HEX  ExportConvexHullGeometry=on  InertiaType=CalculateFromGeometry  BasedOnType=Mass  Density=1000  DensityUnits=kg/m^3  Mass=T_Body_Mass  MassUnits=kg  CenterOfMass=[0 0 0]  CenterOfMassUnits=m  MomentsOfInertia=[1 1 1]  MomentsOfInertiaUnits=kg*m^2  ProductsOfInertia=[0 0 0]  ProductsOfInertiaUnits=kg*m^2  GraphicType=FromGeometry  MarkerShape=Sphere  MarkerSize=10  GraphicVisPropType=SimpleVisualProperties  GraphicDiffuseColor=[0.8 0.0 0.2]  GraphicOpacity=1  GraphicSpecularColor=[0.5 0.5 0.5 1.0]  GraphicAmbientColor=[0.15 0.15 0.15 1.0]  GraphicEmissiveColor=[0.0 0.0 0.0 1.0]  GraphicShininess=75  DoExposeReferenceFrame=on  SerializedFrames=<Frames/>
  Transform Sensor1 : sm_lib/Frames and Transforms/Transform Sensor  MeasurementFrame=Follower  RotationSequence=ZYX  SenseAngle=off  SenseAxis=off  SenseQ=off  SenseR=off  SenseRotationSequence=off  SenseOmegaX=off  SenseOmegaY=off  SenseOmegaZ=off  SenseOmega=on  SenseQDot=off  SenseRDot=off  SenseRotationSequenceDot=off  SenseAlphaX=off  SenseAlphaY=off  SenseAlphaZ=off  SenseAlpha=on  SenseQDDot=off  SenseRDDot=off  SenseX=off  SenseY=off  SenseZ=off  SenseXYZ=off  SenseRad=off  SenseAzim=off  SenseDist=off  SenseInc=off  SenseXDot=off  SenseYDot=off  SenseZDot=off  SenseXYZDot=on  SenseRadDot=off  SenseAzimDot=off  SenseDistDot=off  SenseIncDot=off  SenseXDDot=off  SenseYDDot=off  SenseZDDot=off  SenseXYZDDot=on  SenseRadDDot=off  SenseAzimDDot=off  SenseDistDDot=off  SenseIncDDot=off
  Transform Sensor2 : sm_lib/Frames and Transforms/Transform Sensor  MeasurementFrame=Base  RotationSequence=ZYX  SenseAngle=off  SenseAxis=off  SenseQ=on  SenseR=off  SenseRotationSequence=off  SenseOmegaX=off  SenseOmegaY=off  SenseOmegaZ=off  SenseOmega=on  SenseQDot=off  SenseRDot=off  SenseRotationSequenceDot=off  SenseAlphaX=off  SenseAlphaY=off  SenseAlphaZ=off  SenseAlpha=on  SenseQDDot=off  SenseRDDot=off  SenseX=off  SenseY=off  SenseZ=off  SenseXYZ=on  SenseRad=off  SenseAzim=off  SenseDist=off  SenseInc=off  SenseXDot=off  SenseYDot=off  SenseZDot=off  SenseXYZDot=on  SenseRadDot=off  SenseAzimDot=off  SenseDistDot=off  SenseIncDot=off  SenseXDDot=off  SenseYDDot=off  SenseZDDot=off  SenseXYZDDot=on  SenseRadDDot=off  SenseAzimDDot=off  SenseDistDDot=off  SenseIncDDot=off
  Transform Sensor5 : sm_lib/Frames and Transforms/Transform Sensor  MeasurementFrame=World  RotationSequence=ZYX  SenseAngle=off  SenseAxis=off  SenseQ=on  SenseR=on  SenseRotationSequence=off  SenseOmegaX=off  SenseOmegaY=off  SenseOmegaZ=off  SenseOmega=off  SenseQDot=off  SenseRDot=off  SenseRotationSequenceDot=off  SenseAlphaX=off  SenseAlphaY=off  SenseAlphaZ=off  SenseAlpha=off  SenseQDDot=off  SenseRDDot=off  SenseX=off  SenseY=off  SenseZ=off  SenseXYZ=on  SenseRad=off  SenseAzim=off  SenseDist=off  SenseInc=off  SenseXDot=off  SenseYDot=off  SenseZDot=off  SenseXYZDot=on  SenseRadDot=off  SenseAzimDot=off  SenseDistDot=off  SenseIncDot=off  SenseXDDot=off  SenseYDDot=off  SenseZDDot=off  SenseXYZDDot=on  SenseRadDDot=off  SenseAzimDDot=off  SenseDistDDot=off  SenseIncDDot=off
  World Frame : sm_lib/Frames and Transforms/World Frame
  slip_kinematics : MATLAB Function  TreatAsAtomicUnit=on
  slip_kinematics+Timer : MATLAB Function  TreatAsAtomicUnit=on
  slip_kinematics+Timer1 : MATLAB Function  Commented=on  TreatAsAtomicUnit=on
  slip_kinematics_current : MATLAB Function  TreatAsAtomicUnit=on
  touch : MATLAB Function  TreatAsAtomicUnit=on
  w[deg/sec] : Scope
  wd[deg/s^2] : Scope
  tag scope: S_Acc_wrt_Body=global, S_Acc_wrt_Inertial=global, S_Attitude_quat_Inertial=global, S_Pos_wrt_Inertial=global, S_Rate_wrt_Body=global, S_Rated_wrt_Body=global, S_Vel_wrt_Body=global, S_Vel_wrt_Inertial=global
  wires:
  Radians to Degrees/1 -> Attitude_iner[deg]/1
  Radians to Degrees2/1 -> w[deg/sec]/1
  Quaternions to Rotation Angles/1 -> Radians to Degrees/1
  From2/1 -> Jacobian_based_EE_Control(Rate)/1(q)
  Constant2/1 -> Jacobian_based_EE_Control(Rate)/2(target_pos)
  Constant3/1 -> Fabrik_based_EE_Control(Angle)/1(target)
  Fabrik_based_EE_Control(Angle)/1(q_list) -> Add3/1
  Fabrik_based_EE_Control(Angle)/2(pos_list) -> Display/1
  Jacobian_based_EE_Control(Rate)/1(qd_cmd) -> Gain/1
  Constant4/1 -> Fabrik_based_EE_Control(Angle)/2(tol)
  Constant5/1 -> Fabrik_based_EE_Control(Angle)/3(max_iter)
  MATLAB Function5/1(pos) -> Display1/1
  Fabrik_based_EE_Control(Angle)/3(iter_fin) -> Display6/1
  MATLAB Function6/2(ee_pose) -> Display7/1
  Add3/1 -> MATLAB Function5/1(theta)
  Constant/1 -> Add3/2, Add5/2
  From3/1 -> MATLAB Function2/1(u)
  Constant6/1 -> Degrees to Radians/1
  MATLAB Function2/1(y) -> Display4/1
  Add5/1 -> MATLAB Function6/1(theta)
  From4/1 -> Add5/1
  PS-Simulink Converter23/1 -> [S_Attitude_quat_Inertial]
  PS-Simulink Converter26/1 -> [S_Pos_wrt_Inertial]
  PS-Simulink Converter27/1 -> [S_Vel_wrt_Inertial]
  PS-Simulink Converter28/1 -> [S_Acc_wrt_Inertial]
  PS-Simulink Converter2/1 -> Radians to Degrees3/1, [S_Rated_wrt_Body]
  PS-Simulink Converter1/1 -> Radians to Degrees1/1, [S_Rate_wrt_Body]
  PS-Simulink Converter3/1 -> Scope7/1, [S_Vel_wrt_Body]
  PS-Simulink Converter4/1 -> [S_Acc_wrt_Body], Scope7/2
  Radians to Degrees1/1 -> Scope5/1
  Radians to Degrees3/1 -> Scope5/2
  [S_Attitude_quat_Inertial] -> Quaternions to Rotation Angles/1
  [S_Rate_wrt_Body] -> Radians to Degrees2/1
  [S_Rated_wrt_Body] -> Radians to Degrees4/1
  Radians to Degrees4/1 -> wd[deg/s^2]/1
  Clock1/1 -> Openning_Motion_Sequence1/1(t)
  Constant8/1 -> Subsystem1/5(P_gain)
  [S_Rate_wrt_Body] -> Subsystem1/4(In4)
  Constant9/1 -> Subsystem1/6(I_gain)
  Constant1/1 -> Subsystem1/1(Degrees in)
  Gain2/1 -> Demux1/1
  Subsystem1/1(Omegad) -> Gain2/1
  Pulse Generator/1 -> Subsystem1/Trigger
  Constant7/1 -> Subsystem1/3(In3)
  Constant10/1 -> Subsystem1/7(D_gain)
  PS-Simulink Converter38/1 -> [Service_Body_R]
  Demux1/1 -> Subsystem5/1(RW1_Torque_CMD)
  Demux1/2 -> Subsystem5/2(RW2_Torque_CMD)
  Demux1/3 -> Subsystem5/3(RW3_Torque_CMD)
  Demux1/4 -> Subsystem5/4(RW4_Torque_CMD)
  [Service_Body_R] -> Subsystem5/5(Satellite_Attitude)
  PS-Simulink Converter13/1 -> [Relative_pos]
  PS-Simulink Converter14/1 -> [Relative_Acc]
  PS-Simulink Converter15/1 -> [Relative_Vel]
  PS-Simulink Converter6/1 -> [Relative_wd]
  PS-Simulink Converter5/1 -> [Relative_quat]
  PS-Simulink Converter7/1 -> [Relative_w]
  Quaternions to Rotation Angles1/1 -> Radians to Degrees5/1
  Radians to Degrees5/1 -> Attitude:Rel,Iner/2
  Quaternions to Rotation Angles2/1 -> Radians to Degrees6/1
  Radians to Degrees6/1 -> Attitude:Rel,Iner/1
  [Relative_quat] -> Quaternions to Rotation Angles2/1
  [S_Attitude_quat_Inertial] -> Quaternions to Rotation Angles1/1
  From20/1 -> Scope16/1, Openning_Motion_Sequence4/3(b_flg)
  Gain9/1 -> Scope10/1
  Openning_Motion_Sequence4/1(res) -> Gain9/1
  [Right_ARM_Jt] -> Right_Joint_Torque[Nm]/1
  [S_Attitude_quat_Inertial] -> Subsystem1/2(q)
  [Right_ARM_J] -> Radians to Degrees8/1
  Radians to Degrees8/1 -> Right_Joint_Angle[deg]/1
  [Right_ARM_J] -> End_Position_Flg/1(R_J)
  End_Position_Flg/1(res) -> [Pos_END_FLAG], Display13/1
  From32/1 -> Openning_Motion_Sequence4/4(pos_end_flg)
  Right_ARM_Real_FK/2(ee_pose) -> Display8/1
  Gain8/1 -> Display17/1, Add/1
  Gain7/1 -> Right_ARM_Real_Simple_FK/1(theta)
  MATLAB Function4/1(y) -> Display14/1
  [Right_ARM_J_Vel_Mount] -> MATLAB Function3/1(u)
  Matrix Multiply1/1 -> Scope34/2, [EE_vel_J], Gain8/1
  Right_ARM_Real_Simple_FK/2(ee_pose) -> Scope14/2, Display16/1
  Right_ARM_Jacobian/1(J) -> Matrix Multiply1/1
  [Right_ARM_J_Pos_Mount] -> Scope39/1, MATLAB Function4/1(u)
  [Right_ARM_Jd] -> Matrix Multiply1/2, Scope36/1
  Add/1 -> Matrix 1-Norm/1
  Matrix 1-Norm/1 -> Scope9/1
  Selector/1 -> Add/2
  From9/1 -> Openning_Motion_Sequence4/2(R_J)
  From13/1 -> Openning_Motion_Sequence4/1(R_J_Pos)
  From41/1 -> ?
  Delay2/1 -> Scope37/2, [system_slip_ing]
  Empty/2(joint_current_flg) -> Scope19/1
  [Rv_cmd] -> touch/4(Rv_cmd)
  MATLAB Function11/3(system_slip_confirm) -> Delay3/1
  touch/4(speed_drop_vec) -> Scope31/1
  Sine Wave2/1 -> Multiply2/1
  touch/2(touch_flg) -> [touch_flg], Scope27/1
  MATLAB Function11/4(system_empty) -> Delay4/1
  EE_R/4(RPos_3) -> Display2/1, Derivative1/1, Goto52/1
  touch/3(q_touch_flg) -> Scope26/1
  [slip_confirm_flg] -> MATLAB Function11/2(slip_confirm_flg)
  Derivative1/1 -> Scope8/1
  Delay3/1 -> Scope37/3, [system_slip_confirm]
  [empty_flg] -> MATLAB Function11/5(empty_flg)
  [Right_ARM_J_Pos_SB] -> Gain1/1
  Slip_current/3(I_avg_now) -> Scope24/1
  Slip_current/1(slip_warning_flg) -> Scope1/1, [slip_warning_flg]
  [touch_flg] -> MATLAB Function11/4(touch_flg)
  Slip_current/5(dI_flg) -> Scope29/1
  EE_R/3(RPos_2) -> Scope18/1, Goto51/1
  EE_R/1(RPos_0) -> Goto49/1
  MATLAB Function11/1(system_overload) -> Delay1/1
  [Right_ARM_Jd] -> touch/3(R_Jd)
  [touch_start] -> touch/1(touch_start)
  EE_R/2(RPos_1) -> Goto50/1
  Slip_current/6(abs_I_flg) -> Scope29/2
  Slip_current/2(slip_confirm_flg) -> [slip_confirm_flg], Scope25/1
  Delay1/1 -> Scope37/1, [system_overload]
  [slip_warning_flg] -> MATLAB Function11/1(slip_warning_flg)
  [touch_flg] -> Slip_current/2(touch_flg)
  [overload_start] -> Overload/2(overload_start)
  From102/1 -> EE_R/1(R_J)
  [Right_ARM_Jt] -> Slip_current/1(R_jtc)
  [Right_ARM_Jt] -> Empty/2(R_jtc)
  Empty/1(empty_flg) -> [empty_flg], Scope2/1
  [Right_ARM_Jt] -> touch/2(R_jtc)
  Delay4/1 -> Scope37/4, [system_empty]
  [OVerload_flg] -> MATLAB Function11/3(Overload_flg)
  touch/1(speed_drop_flg) -> Scope13/1
  [Right_ARM_Jt] -> Overload/1(R_jtc)
  Overload/1(overload_flg) -> Scope6/1, [OVerload_flg]
  MATLAB Function11/2(system_slip_ing) -> Delay2/1
  Slip_current/4(dI) -> Scope28/1
  Gain1/1 -> Submatrix/1, Empty/1(RPos_3)
  Empty/3(RPos) -> Scope4/1
  Sine Wave3/1 -> Multiply3/1
  Sine Wave4/1 -> Multiply4/1
  Sine Wave/1 -> Multiply/1
  Sine Wave1/1 -> Multiply1/1
  Clock/1 -> MATLAB Function16/4(elapsedTime)
  [Right_ARM_J_Pos_SB] -> Gain3/1
  Gain3/1 -> MATLAB Function16/2(R_J_Pos)
  [Right_ARM_J] -> MATLAB Function16/1(R_J)
  Radians to Degrees7/1 -> MATLAB Function16/3(R_q)
  [Right_ARM_J] -> Radians to Degrees7/1
  Submatrix/1 -> Scope3/1
  MATLAB Function16/1(Z) -> Scope/1
  MATLAB Function16/2(control_mode) -> [control_mode], Scope11/1
  MATLAB Function16/3(Rv_cmd) -> Scope20/1, [Rv_cmd]
  MATLAB Function16/4(flag_empty_now) -> Scope12/1
  MATLAB Function16/5(touch_start) -> [touch_start]
  MATLAB Function16/6(overload_start) -> [overload_start]
  MATLAB Function16/8(Body_contact) -> Scope15/1
  [system_empty] -> MATLAB Function16/9(system_empty)
  [Rv_cmd] -> Right_ARM/1(J_cmd)
  [control_mode] -> Right_ARM/2(Mode)
  [Right_ARM_J_Pos_SB] -> Gain4/1
  Gain4/1 -> Submatrix1/1
  [system_slip_ing] -> MATLAB Function16/11(system_slip_ing)
  [system_slip_confirm] -> Scope35/1, MATLAB Function16/12(system_slip_confirm)
  [B_f1_contact] -> MATLAB Function16/5(Body_f1)
  [B_f2_contact] -> MATLAB Function16/6(Body_f2)
  [B_f4_contact] -> MATLAB Function16/8(Body_f4)
  [B_f3_contact] -> MATLAB Function16/7(Body_f3)
  [system_overload] -> MATLAB Function16/10(system_overload)
  Submatrix1/1 -> Derivative/1, Scope17/1, MATLAB Function11/6(RPos_3)
  Derivative/1 -> Scope32/1
  MATLAB Function3/1(y) -> Scope33/1, Display18/1, Selector/1
  [Right_ARM_J] -> Derivative3/1, Scope40/1, Right_ARM_Jacobian/1(theta), Right_ARM_Real_FK/1(theta), Gain7/1
  Derivative3/1 -> Scope38/1
  [Right_ARM_J_Pos_Mount] -> MATLAB Function1/1(u), Display3/1
  MATLAB Function1/1(y) -> Derivative4/1
  Derivative4/1 -> Scope21/1
  [EE_vel_J] -> slip_kinematics/1(EE_vel_J), Delay/1
  slip_kinematics/2(slip_kinematics) -> [slip_kine_flg], Scope22/1
  Delay/1 -> slip_kinematics/2(EE_vel_J_pre)
  slip_kinematics/1(EE_vel_t) -> Scope23/1
  MATLAB Function16/7(EE_Jaco_start) -> [EE_Jaco_start]
  [EE_Jaco_start] -> slip_kinematics/3(EE_Jaco_start)
  [slip_kine_flg] -> slip_kinematics_current/1(slip_kine_flg)
  [slip_warning_flg] -> slip_kinematics_current/2(slip_warning_flg)
  slip_kinematics_current/1(slip_dual_flg) -> [slip_dual_flg], Scope30/1
  [slip_dual_flg] -> Delay5/1
  Delay5/1 -> slip_kinematics_current/3(slip_dual_flg_pre)
  Clock2/1 -> MATLAB Function/1(elapsedTime)
  MATLAB Function/2(differ_input) -> Scope43/1
  slip_kinematics+Timer/1(EE_vel_t) -> Scope42/1
  slip_kinematics+Timer/2(slip_kinematics) -> Scope41/1
  [EE_Jaco_start] -> slip_kinematics+Timer/2(EE_Jaco_start)
  [EE_vel_J] -> Scope45/1, slip_kinematics+Timer/1(EE_vel_J)
  Clock3/1 -> slip_kinematics+Timer/3(elapsedTime)
  Clock4/1 -> slip_kinematics+Timer1/3(elapsedTime)
  From78/1 -> slip_kinematics+Timer1/2(EE_Jaco_start)
  slip_kinematics+Timer1/2(slip_kinematics) -> Scope46/1
  slip_kinematics+Timer1/1(EE_vel_t) -> Scope47/1
  From79/1 -> Scope48/1, slip_kinematics+Timer1/1(EE_vel_J)
  MATLAB Function/1(dTime) -> Scope49/1
  MATLAB Function7/1(dTime) -> Scope51/1
  Ramp2/1 -> MATLAB Function7/2(input)
  MATLAB Function7/2(differ_input) -> Scope50/1
  Clock5/1 -> MATLAB Function7/1(elapsedTime)
  Sine Wave5/1 -> Scope44/1, MATLAB Function/2(input)
  [EE_vel_J] -> Scope54/1, Subsystem/1(u)
  Subsystem/1(y) -> Scope52/1
  Pulse Generator1/1 -> Subsystem/Trigger, Scope53/1
  connections:
  Spatial Contact Force6/RConn1 -- Target/LConn1 -- Right_ARM/LConn4 -- Subsystem2/RConn2
  Transform Sensor5/RConn1 -- Transform Sensor2/LConn1 -- Brick Solid/RConn2 -- Right_ARM/LConn2 -- Transform Sensor1/RConn1
  6-DOF Joint2/LConn1 -- World Frame/RConn1 -- Mechanism Configuration/RConn1 -- 6-DOF Joint3/LConn1 -- 6-DOF Joint1/LConn1 -- Solver Configuration/RConn1
  6-DOF Joint1/RConn1 -- 6-DOF Joint3/RConn1 -- Target/RConn1 -- Transform Sensor2/RConn1
  Brick Solid/RConn1 -- 6-DOF Joint2/RConn1
  Transform Sensor1/RConn3 -- PS-Simulink Converter2/LConn1
  Transform Sensor1/RConn2 -- PS-Simulink Converter1/LConn1
  Transform Sensor1/RConn4 -- PS-Simulink Converter3/LConn1
  Transform Sensor1/RConn5 -- PS-Simulink Converter4/LConn1
  Transform Sensor5/RConn6 -- PS-Simulink Converter28/LConn1
  Transform Sensor5/RConn5 -- PS-Simulink Converter27/LConn1
  Transform Sensor5/RConn4 -- PS-Simulink Converter26/LConn1
  Transform Sensor5/RConn2 -- PS-Simulink Converter23/LConn1
  Transform Sensor5/RConn3 -- PS-Simulink Converter38/LConn1
  Spatial Contact Force6/LConn1 -- Brick Solid/RConn3 -- Right_ARM/LConn3
  Transform Sensor2/RConn5 -- PS-Simulink Converter13/LConn1
  Transform Sensor2/RConn6 -- PS-Simulink Converter15/LConn1
  Transform Sensor2/RConn7 -- PS-Simulink Converter14/LConn1
  PS-Simulink Converter5/LConn1 -- Transform Sensor2/RConn2
  Transform Sensor2/RConn3 -- PS-Simulink Converter7/LConn1
  Transform Sensor2/RConn4 -- PS-Simulink Converter6/LConn1
  Brick Solid/LConn3 -- Subsystem2/RConn1
  Brick Solid/LConn1 -- Right_ARM/LConn1
  Brick Solid/LConn2 -- Subsystem5/LConn1
